simulink model "PI_Regler_LABOR_Thu"  (R2018a)
settings: Solver=FixedStepAuto  StartTime=0.0  StopTime=3  FixedStep=1e-5  RelTol=1e-3  EnableMultiTasking=on
values from neighbouring files (symbols this model uses):
  Cr = 7.2352*10^-6    (= 7.2352e-06)    [lab04_part01.m]    (also in lab05_part01_baga.m; lab06_simulationWithMeasurements.m)
  J = 5.5e-6    (= 5.5e-06)    [lab03_part01.m]    (also in lab04_part01.m = 8e-06; lab05_part01_baga.m = 8e-06; lab06_simulationWithMeasurements.m = 5.29e-06)
  k_e = 23.7e-3    (= 0.0237)    [lab03_part01.m]    (also in lab06_simulationWithMeasurements.m = 0.02375)
  k_i = (w_0*w_0 * J * R_A) / k_m    (= 0.474003784506)    [lab06_simulationWithMeasurements.m]
  k_m = 22.46e-3    (= 0.02246)    [lab03_part01.m]    (also in lab06_simulationWithMeasurements.m)
  k_p = (2 * D * w_0 * J * R_A - k_e * k_m- R_A * Cr) / k_m    (= 0.00175693036509)    [lab06_simulationWithMeasurements.m]
  L = tan(phi).*Rges./(frequencies.*2*pi)    [lab02_part01.m]    (also in lab03_part01.m = 0.0005752; lab04_part01.m = 0.00035329; lab05_part01_baga.m = 0.00035329; lab06_simulationWithMeasurements.m = 0.000618)
  R_A = 3.22    [lab03_part01.m]    (also in lab05_part01_baga.m = 3.71; lab06_simulationWithMeasurements.m)
  R_S = 1    [lab03_part01.m]    (also in lab05_part01_baga.m; lab06_simulationWithMeasurements.m)
  w_soll = 450    [lab05_part01_baga.m]    (also in lab06_simulationWithMeasurements.m = 250)
settings Model: Creator=Felix  LastModifiedBy=oleksandra
settings OptimizationCC: LifeSpan=inf
settings DebuggingCC: SFUnexpectedBacktrackingDiag=warning  SFNoUnconditionalDefaultTransitionDiag=warning  SFExecutionAtInitializationDiag=none
settings CodeAppCC: StateflowObjectComments=on
settings GRTTargetCC: TargetLangStandard=C89/C90 (ANSI)  GeneratePreprocessorConditionals=Disable all
settings ConfigComp: CovMetricSettings=dw  CovHtmlReporting=on  CovSaveCumulativeToWorkspaceVar=on  CovSaveSingleToWorkspaceVar=on  CovExternalEMLEnable=off

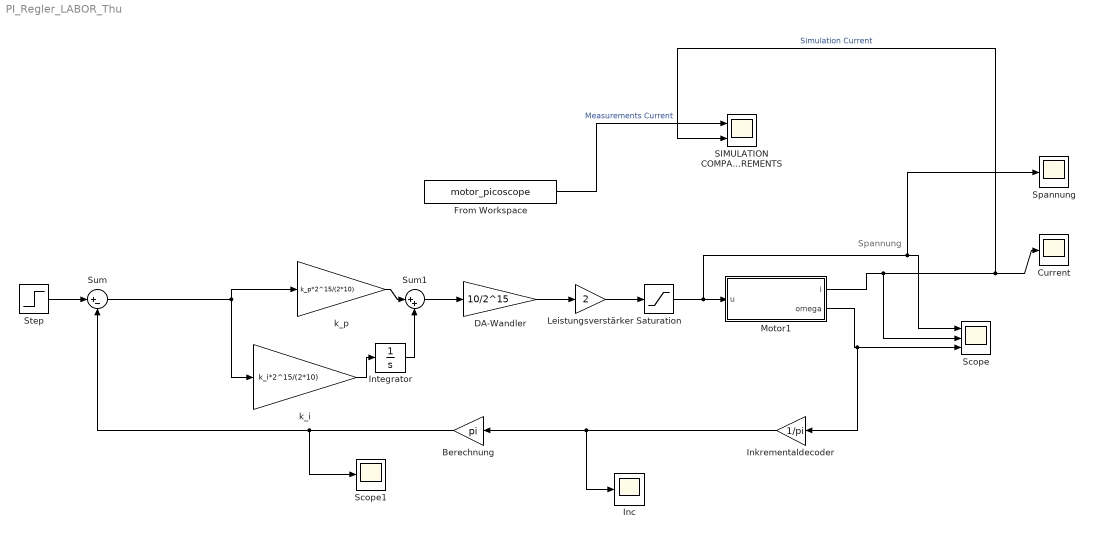
== system PI_Regler_LABOR_Thu ==
  note: Spannung
  Berechnung : Gain  Gain=pi
  Current : Scope
  DA-Wandler : Gain  Gain=10/2^15
  From Workspace : FromWorkspace  VariableName=motor_picoscope
  Inc : Scope
  Inkrementaldecoder : Gain  Gain=1/pi
  Integrator : Integrator
  Leistungsverstärker : Gain  Gain=2
  Motor1 : Subsystem  TreatAsAtomicUnit=on
  SIMULATION COMPARED TO MEASUREMENTS : Scope  NumInputPorts=2
  Saturation : Saturate  UpperLimit=12  LowerLimit=-12
  Scope : Scope  NumInputPorts=3
  Scope1 : Scope
  Spannung : Scope
  Step : Step  After=w_soll  SampleTime=0
  Sum : Sum  Inputs=|+-
  Sum1 : Sum  Inputs=|++
  k_i : Gain  Gain=k_i*2^15/(2*10)
  k_p : Gain  Gain=k_p*2^15/(2*10)
  wires:
  Leistungsverstärker/1 -> Saturation/1
  DA-Wandler/1 -> Leistungsverstärker/1
  Step/1 -> Sum/1
  Saturation/1 -> Motor1/1(u), Spannung/1, Scope/1
  k_i/1 -> Integrator/1
  k_p/1 -> Sum1/1
  Sum1/1 -> DA-Wandler/1
  Integrator/1 -> Sum1/2
  Inkrementaldecoder/1 -> Inc/1, Berechnung/1
  Berechnung/1 -> Scope1/1, Sum/2
  Sum/1 -> k_i/1, k_p/1
  Motor1/1(i) -> Scope/2, SIMULATION COMPARED TO MEASUREMENTS/2, Current/1  "Simulation Current"
  Motor1/2(omega) -> Inkrementaldecoder/1, Scope/3
  From Workspace/1 -> SIMULATION COMPARED TO MEASUREMENTS/1  "Measurements Current"

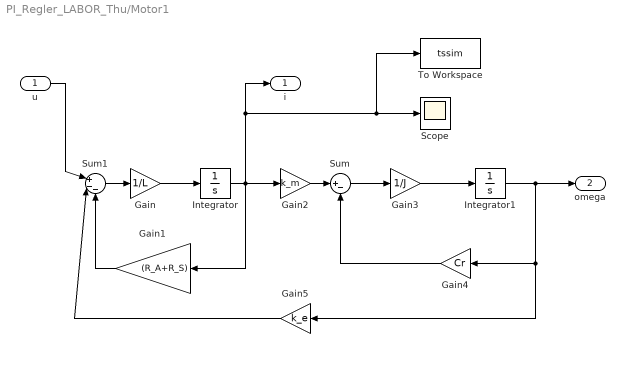
== system PI_Regler_LABOR_Thu/Motor1 ==
  u : Inport
  Gain : Gain  Gain=1/L  SaturateOnIntegerOverflow=on  OutDataTypeStr=Inherit: Same as input  ParamDataTypeStr=Inherit: Same as input
  Gain1 : Gain  Gain=(R_A+R_S)  SaturateOnIntegerOverflow=on  OutDataTypeStr=Inherit: Same as input  ParamDataTypeStr=Inherit: Same as input
  Gain2 : Gain  Gain=k_m  SaturateOnIntegerOverflow=on  OutDataTypeStr=Inherit: Same as input  ParamDataTypeStr=Inherit: Same as input
  Gain3 : Gain  Gain=1/J  SaturateOnIntegerOverflow=on  OutDataTypeStr=Inherit: Same as input  ParamDataTypeStr=Inherit: Same as input
  Gain4 : Gain  Gain=Cr  SaturateOnIntegerOverflow=on  OutDataTypeStr=Inherit: Same as input  ParamDataTypeStr=Inherit: Same as input
  Gain5 : Gain  Gain=k_e  SaturateOnIntegerOverflow=on  OutDataTypeStr=Inherit: Same as input  ParamDataTypeStr=Inherit: Same as input
  Integrator : Integrator
  Integrator1 : Integrator
  Scope : Scope
  Sum : Sum  Inputs=|+-  SaturateOnIntegerOverflow=on  InputSameDT=on  OutDataTypeStr=Inherit: Same as first input
  Sum1 : Sum  Inputs=|+--  SaturateOnIntegerOverflow=on  InputSameDT=on  OutDataTypeStr=Inherit: Same as first input
  To Workspace : ToWorkspace  VariableName=tssim  SaveFormat=Timeseries  SampleTime=-1
  i : Outport  Unit=A
  omega : Outport  Port=2  Unit=1/s
  wires:
  Sum1/1 -> Gain/1
  Gain/1 -> Integrator/1
  Gain2/1 -> Sum/1
  Sum/1 -> Gain3/1
  Gain3/1 -> Integrator1/1
  Gain1/1 -> Sum1/3
  Gain4/1 -> Sum/2
  Integrator1/1 -> omega/1, Gain4/1, Gain5/1
  Gain5/1 -> Sum1/2
  Integrator/1 -> To Workspace/1, Scope/1, i/1, Gain2/1, Gain1/1
  u/1 -> Sum1/1
